simulink model "inverter"  (R2024a)
settings: Solver=ode113  StartTime=0  StopTime=5  FixedStep=1e-5  RelTol=1e-3
libraries: simulink x7, spsIGBTDiodeLib x6, spsThreePhaseSeriesRLCBranchLib x3, spsGroundLib x2, spsDCVoltageSourceLib x1, spsThreePhaseVIMeasurementLib x1, sps_lib x1
settings Model: Creator=ammarabdulrasheed  LastModifiedBy=ammarabdulrasheed
settings DataIOCC: ReturnWorkspaceOutputs=off

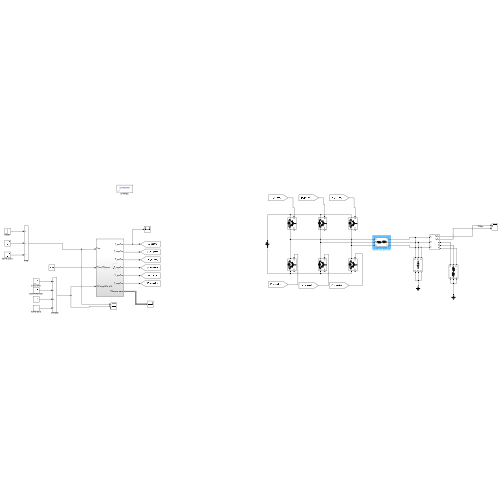
[thumbnail: Simulink's stored preview of the top-level diagram]
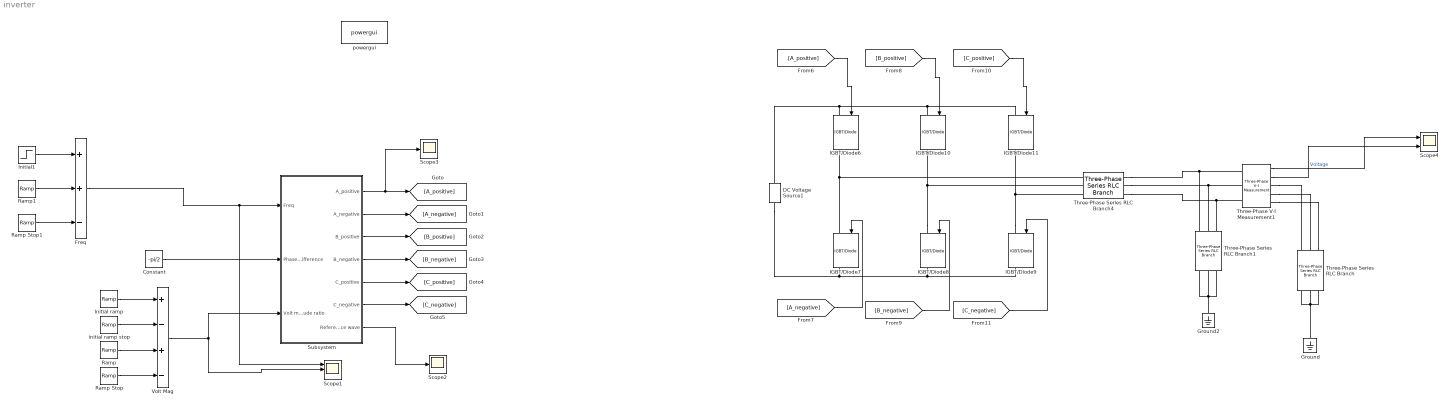
== system inverter ==
  Constant : Constant  Value=-pi/2
  DC Voltage Source1 : spsDCVoltageSourceLib/DC Voltage Source  Amplitude=200  Measurements=None
  Freq : Sum  Inputs=++-
  Ground : spsGroundLib/Ground  LConnTagsString=a
  Ground2 : spsGroundLib/Ground  LConnTagsString=a
  IGBT/Diode{6..11} (6 alike) : spsIGBTDiodeLib/IGBT//Diode  Ron=1e-3  Rs=1e5  Cs=inf  Measurements=on
  Initial ramp : simulink/Sources/Ramp  slope=0.08  start=0  InitialOutput=0
  Initial1 : Step  Time=0  After=0  SampleTime=0
  Ramp : simulink/Sources/Ramp  slope=25*(0.8/50)  start=1 + (0.08/0.8)  InitialOutput=0.04
  Ramp Stop : simulink/Sources/Ramp  slope=25*(0.8/50)  start=3  InitialOutput=0
  Ramp Stop1 : simulink/Sources/Ramp  slope=25  start=3  InitialOutput=0
  Ramp1 : simulink/Sources/Ramp  slope=25  start=1  InitialOutput=0
  Scope1 : Scope  NumInputPorts=3
  Scope2 : Scope
  Scope3 : Scope
  Scope4 : Scope  NumInputPorts=2
  Subsystem : Subsystem
  Three-Phase Series RLC Branch : spsThreePhaseSeriesRLCBranchLib/Three-Phase Series RLC Branch  LConnTagsString=A|B|C  RConnTagsString=A|B|C  BranchType=RL  Resistance=2  Inductance=90e-3  Capacitance=1e-6  Measurements=None
  Three-Phase Series RLC Branch1 : spsThreePhaseSeriesRLCBranchLib/Three-Phase Series RLC Branch  LConnTagsString=A|B|C  RConnTagsString=A|B|C  BranchType=C  Resistance=1e-6  Inductance=1e-3  Capacitance=250e-6  Measurements=None
  Three-Phase Series RLC Branch4 : spsThreePhaseSeriesRLCBranchLib/Three-Phase Series RLC Branch  LConnTagsString=A|B|C  RConnTagsString=A|B|C  BranchType=RL  Resistance=2  Inductance=10e-3  Capacitance=1e-6  Measurements=None
  Three-Phase V-I Measurement1 : spsThreePhaseVIMeasurementLib/Three-Phase V-I Measurement  VoltageMeasurement=phase-to-ground  SetLabelV=off  LabelV=Vabc  Vpu=off  VpuLL=off  CurrentMeasurement=yes  SetLabelI=off  LabelI=Iabc  Ipu=off  Pbase=100e6  Vbase=500e3  OutputType=Complex  PhasorSimulation=off  PSBequivalent=0
  Volt Mag : Sum  Inputs=+-+-
  initial ramp stop : simulink/Sources/Ramp  slope=0.08  start=0.5  InitialOutput=0
  powergui : sps_lib/powergui  Priority=1  SimulationMode=Continuous  SampleTime=50e-6  frequency=60  Iterations=50  frequencyindice=0  Pbase=100e6  ErrMax=1e-4  UnitsV=kV  UnitsW=MW  buscounter=0  FunctionMessages=off  echomessages=off  EnableUseOfTLC=off  CurrentSourceSwitches=off  DisableSnubberDevices=off  DisableRonSwitches=off  DisableVfSwitches=off  DisplayEquations=off  AutomaticDiscreteSolvers=off  SolverType=Tustin/Backward Euler (TBE)  Interpol=off  ExternalGateDelay=off  methode=off  Ts=100  x0status=blocks  SPID=on  SwTol=0  HookPort=off  NonlinearTolerance=1e-4  nMaxIteration=100  ContinueOnMaxIteration=off  RestoreLinks=warning  ResistiveCurrentMeasurement=off  Frange=[0:2:500]  Ylog=off  Xlog=on  ShowGrid=off  save=off  variable=ZData  structure=0  ZoomFFT=off  StartTime=0.0  cycles=1  DisplayStyle=1  fundamental=60  FreqAxis=off  MaxFrequency=1000  frequencyindicesteady=1  RmsSteady=1  display=off
  wires:
  Initial ramp/1 -> Volt Mag/1
  Ramp Stop/1 -> Volt Mag/4
  initial ramp stop/1 -> Volt Mag/2
  Ramp/1 -> Volt Mag/3
  Initial1/1 -> Freq/1
  Constant/1 -> Subsystem/2(Phase Difference)
  Subsystem/1(A_positive) -> Scope3/1, [A_positive]
  Subsystem/2(A_negative) -> [A_negative]
  Subsystem/3(B_positive) -> [B_positive]
  Subsystem/4(B_negative) -> [B_negative]
  Subsystem/5(C_positive) -> [C_positive]
  Subsystem/6(C_negative) -> [C_negative]
  Subsystem/7(Reference wave) -> Scope2/1
  [A_positive] -> IGBT/Diode6/1
  [B_positive] -> IGBT/Diode10/1
  [B_negative] -> IGBT/Diode8/1
  [A_negative] -> IGBT/Diode7/1
  [C_positive] -> IGBT/Diode11/1
  [C_negative] -> IGBT/Diode9/1
  Three-Phase V-I Measurement1/1 -> Scope4/1  "Voltage"
  Three-Phase V-I Measurement1/2 -> Scope4/2
  Ramp1/1 -> Freq/2
  Ramp Stop1/1 -> Freq/3
  Freq/1 -> Scope1/1, Subsystem/1(Freq)
  Volt Mag/1 -> Subsystem/3(Volt magnitude ratio), Scope1/2
  connections:
  IGBT/Diode6/LConn1 -- DC Voltage Source1/RConn1 -- IGBT/Diode11/LConn1 -- IGBT/Diode10/LConn1
  IGBT/Diode7/RConn1 -- DC Voltage Source1/LConn1 -- IGBT/Diode9/RConn1 -- IGBT/Diode8/RConn1
  IGBT/Diode8/LConn1 -- Three-Phase Series RLC Branch4/LConn2 -- IGBT/Diode10/RConn1
  Three-Phase Series RLC Branch4/RConn1 -- Three-Phase Series RLC Branch1/LConn1 -- Three-Phase V-I Measurement1/LConn1
  Three-Phase Series RLC Branch4/RConn3 -- Three-Phase Series RLC Branch1/LConn3 -- Three-Phase V-I Measurement1/LConn3
  IGBT/Diode9/LConn1 -- Three-Phase Series RLC Branch4/LConn3 -- IGBT/Diode11/RConn1
  Three-Phase Series RLC Branch4/RConn2 -- Three-Phase Series RLC Branch1/LConn2 -- Three-Phase V-I Measurement1/LConn2
  IGBT/Diode6/RConn1 -- Three-Phase Series RLC Branch4/LConn1 -- IGBT/Diode7/LConn1
  Three-Phase Series RLC Branch/RConn2 -- Ground/LConn1 -- Three-Phase Series RLC Branch/RConn1 -- Three-Phase Series RLC Branch/RConn3
  Three-Phase V-I Measurement1/RConn3 -- Three-Phase Series RLC Branch/LConn3
  Three-Phase V-I Measurement1/RConn2 -- Three-Phase Series RLC Branch/LConn2
  Three-Phase V-I Measurement1/RConn1 -- Three-Phase Series RLC Branch/LConn1
  Three-Phase Series RLC Branch1/RConn1 -- Three-Phase Series RLC Branch1/RConn2 -- Ground2/LConn1 -- Three-Phase Series RLC Branch1/RConn3

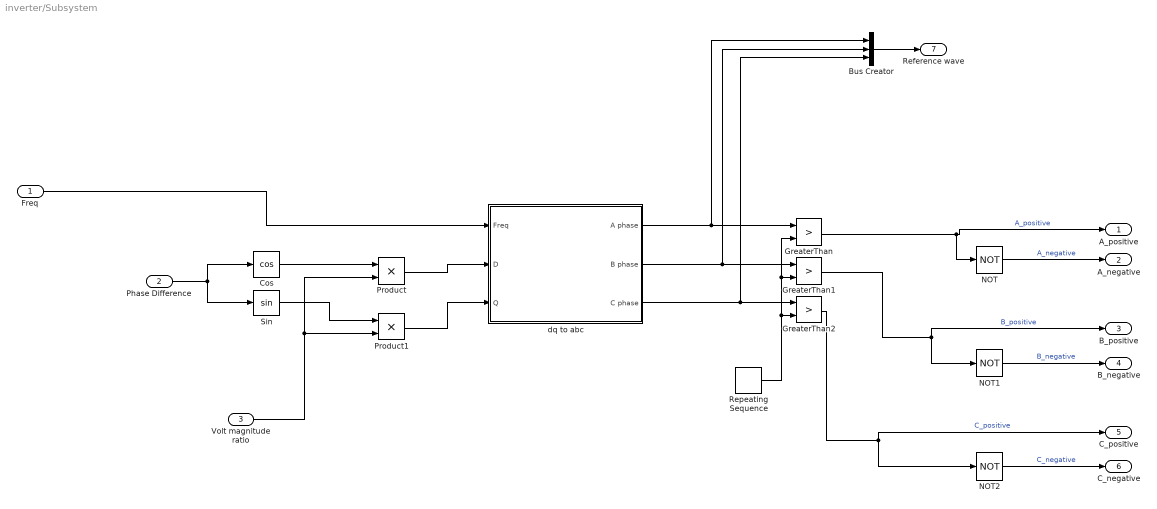
== system inverter/Subsystem ==
  Freq : Inport
  Phase Difference : Inport  Port=2
  Volt magnitude ratio : Inport  Port=3
  Bus Creator : BusCreator  Inputs=3
  Cos : Trigonometry  Operator=cos
  GreaterThan : RelationalOperator  Operator=>  OutDataTypeStr=boolean  RndMeth=Simplest  InputSameDT=off
  GreaterThan1 : RelationalOperator  Operator=>  OutDataTypeStr=boolean  RndMeth=Simplest  InputSameDT=off
  GreaterThan2 : RelationalOperator  Operator=>  OutDataTypeStr=boolean  RndMeth=Simplest  InputSameDT=off
  NOT : Logic  Operator=NOT  IconShape=distinctive  AllPortsSameDT=off  OutDataTypeStr=boolean
  NOT1 : Logic  Operator=NOT  IconShape=distinctive  AllPortsSameDT=off  OutDataTypeStr=boolean
  NOT2 : Logic  Operator=NOT  IconShape=distinctive  AllPortsSameDT=off  OutDataTypeStr=boolean
  Product : Product
  Product1 : Product
  Repeating Sequence : simulink/Sources/Repeating Sequence  rep_seq_t=[0 1 2 3 4]*(1/5)*0.5e-3  rep_seq_y=[0 1 0 -1 0]
  Sin : Trigonometry
  dq to abc : Subsystem
  A_positive : Outport
  A_negative : Outport  Port=2
  B_positive : Outport  Port=3
  B_negative : Outport  Port=4
  C_positive : Outport  Port=5
  C_negative : Outport  Port=6
  Reference wave : Outport  Port=7
  wires:
  NOT2/1 -> C_negative/1  "C_negative"
  Product1/1 -> dq to abc/3(Q)
  Phase Difference/1 -> Sin/1, Cos/1
  NOT1/1 -> B_negative/1  "B_negative"
  Repeating Sequence/1 -> GreaterThan/2, GreaterThan1/2, GreaterThan2/2
  Sin/1 -> Product1/1
  Volt magnitude ratio/1 -> Product1/2, Product/2
  Cos/1 -> Product/1
  NOT/1 -> A_negative/1  "A_negative"
  GreaterThan/1 -> A_positive/1, NOT/1  "A_positive"
  GreaterThan1/1 -> B_positive/1, NOT1/1  "B_positive"
  GreaterThan2/1 -> C_positive/1, NOT2/1  "C_positive"
  Product/1 -> dq to abc/2(D)
  dq to abc/2(B phase) -> Bus Creator/2, GreaterThan1/1
  dq to abc/3(C phase) -> Bus Creator/3, GreaterThan2/1
  Freq/1 -> dq to abc/1(Freq)
  dq to abc/1(A phase) -> Bus Creator/1, GreaterThan/1
  Bus Creator/1 -> Reference wave/1

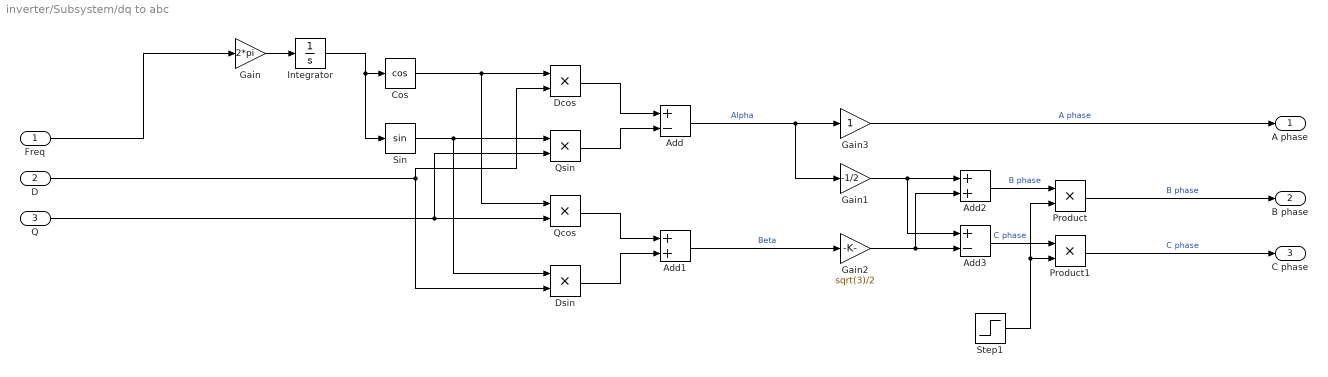
== system inverter/Subsystem/dq to abc ==
  Freq : Inport
  D : Inport  Port=2
  Q : Inport  Port=3
  Add : Sum  Inputs=+-
  Add1 : Sum
  Add2 : Sum
  Add3 : Sum  Inputs=+-
  Cos : Trigonometry  Operator=cos
  Dcos : Product
  Dsin : Product
  Gain : Gain  Gain=2*pi
  Gain1 : Gain  Gain=-1/2
  Gain2 : Gain  Gain=sqrt(3)/2
  Gain3 : Gain
  Integrator : Integrator
  Product : Product
  Product1 : Product
  Qcos : Product
  Qsin : Product
  Sin : Trigonometry
  Step1 : Step  Time=0  SampleTime=0
  A phase : Outport
  B phase : Outport  Port=2
  C phase : Outport  Port=3
  wires:
  Product/1 -> B phase/1  "B phase"
  Add1/1 -> Gain2/1  "Beta"
  Product1/1 -> C phase/1  "C phase"
  D/1 -> Dsin/2, Dcos/2
  Dsin/1 -> Add1/2
  Freq/1 -> Gain/1
  Step1/1 -> Product1/2, Product/2
  Q/1 -> Qcos/2, Qsin/2
  Dcos/1 -> Add/1
  Gain/1 -> Integrator/1
  Gain3/1 -> A phase/1  "A phase"
  Cos/1 -> Qcos/1, Dcos/1
  Add2/1 -> Product/1  "B phase"
  Gain2/1 -> Add3/2, Add2/2
  Integrator/1 -> Sin/1, Cos/1
  Add3/1 -> Product1/1  "C phase"
  Sin/1 -> Dsin/1, Qsin/1
  Gain1/1 -> Add3/1, Add2/1
  Qsin/1 -> Add/2
  Qcos/1 -> Add1/1
  Add/1 -> Gain1/1, Gain3/1  "Alpha"
